simulink model "UNICO_simulink"  (R2023a)
settings: Solver=FixedStepAuto  StartTime=0.0  StopTime=750  RelTol=1e-3
undefined symbols (not defined in the file): Control, OutList, strmatch
libraries: cstblocks x3, simulink x2
settings Model: Creator=emanu  LastModifiedBy=utente
settings SolverCC: ZeroCrossAlgorithm=Adaptive
settings OptimizationCC: ReuseModelBlockBuffer=off
settings DebuggingCC: MaxConsecutiveZCsMsg=warning  IgnoredZcDiagnostic=none
settings ModelReferenceCC: EnableRefExpFcnMdlSchedulingChecks=on
settings RTWCC: Description=Create Visual C/C++ Solution File for Simulink Coder  SystemTargetFile=discon.tlc  TemplateMakefile=discon_vc.tmf
settings GRTTargetCC: UseToolchainInfoCompliant=off

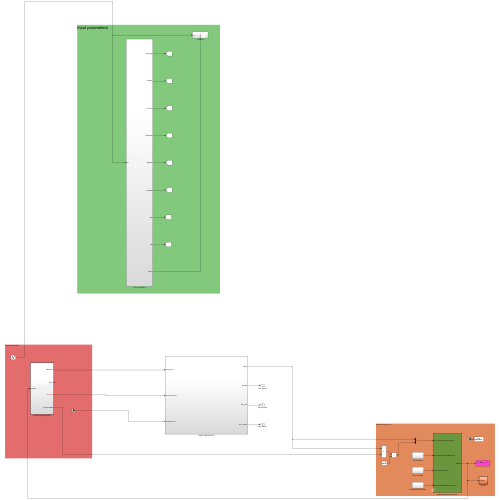
[thumbnail: Simulink's stored preview of the top-level diagram]
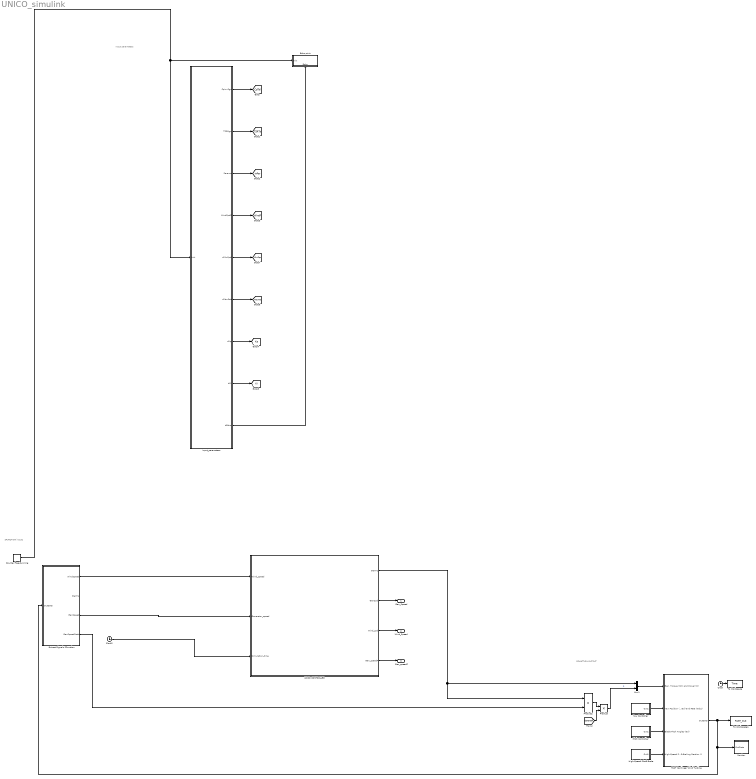
== system UNICO_simulink ==
  note: SFUNCTION inputs
  note: SFUNCTION OUTPUT
  note: Input parameters
  Clock : Clock
  Clock2 : Clock
  Counter Free-Running : simulink/Sources/Counter Free-Running  NumBits=64  tsamp=-1
  Echo print : Subsystem
      settings: PortSchema="{\"entries\":[{\"content\":{\"sides\":[{\"content\":{\"connectorIds\":[\"In1\"]},\"type\":\"ConnectorPlacement.EquallySpacedRectSide\",\"uuid\":\"a7404841-4279-4901-8e4b-4d9f651fd70d\"},{\"content\":{\"side\":\"RIGHT\"},\"type\":\"ConnectorPlacement.EquallySpacedRectSide\",\"uuid\":\"c083252d-994d-448b-85dd-b05fa098362a\"},{\"content\":{\"connectorIds\":[\"In2\"],\"side\":\"TOP\"},\"type\":\"ConnectorPlacement.EquallySpacedRectSide\",\"uuid\":\"2158789e-5709-45dd-87ec-c3c83921db3a\"}]},\"type\":\"ConnectorPlacement.EquallySpacedConnector\",\"uuid\":\"2f3f8f4d-3210-4d41-988d-02cc8661526f\"}],\"packageUris\":[\"http://schema.mathworks.com/mf0/Connector/R2020b\"],\"version\":\"1.0\"}"
  Extract Signals SFunction : Subsystem  TreatAsAtomicUnit=on
  FAST Nonlinear Wind Turbine : Subsystem  mask(FAST Nonlinear Wind Turbine){}
      mask help: This block contains the FAST S-Function.
      mask init:
      | clear FAST_SFunc
  High-Speed Shaft Brake : Subsystem
  Input_parameters : Subsystem
  Monitor : Subsystem  TreatAsAtomicUnit=on
  Mux1 : Mux  Inputs=2
  Pitch Controller : Subsystem
  Product : Product
  Product2 : Product
  To Workspace : ToWorkspace  VariableName=Time  SampleTime=-1
  To Workspace1 : ToWorkspace  VariableName=FAST_Out  SaveFormat=Timeseries  SampleTime=-1
  UNICO CONTROLLER : Subsystem
  Yaw Controller : Subsystem
  Gen_Speed : Outport
  Wind_Speed : Outport  Port=2
  Gen_speedF : Outport  Port=3
  tag scope: CpTbl=global, InPar=global, Ki=global, Kp=global, MaxRat=global, MinSpd=global, TSRTb=global, WindF=global
  wires:
  Pitch Controller/1(Out1) -> FAST Nonlinear Wind Turbine/3(Blade Pitch Angles (rad))
  High-Speed Shaft Brake/1(Out1) -> FAST Nonlinear Wind Turbine/4(High-Speed Shaft Braking Fraction (-))
  FAST Nonlinear Wind Turbine/1(OutData) -> Extract Signals SFunction/1(OutData), Monitor/1(OutData), To Workspace1/1
  Clock/1 -> To Workspace/1
  Yaw Controller/1(Out1) -> FAST Nonlinear Wind Turbine/2(Yaw Position (rad) and Rate (rad/s))
  Clock2/1 -> UNICO CONTROLLER/3(Simulation_time)
  Mux1/1 -> FAST Nonlinear Wind Turbine/1(Gen. Torque (Nm) and Power (W))
  Product2/1 -> Product/1
  Product/1 -> Mux1/2  "P"
  Input_parameters/9(dEcho) -> Echo print/2(Echo)
  Counter Free-Running/1 -> Echo print/1(Init), Input_parameters/1(Init)
  Input_parameters/2(TSRSgn) -> [TSRTb]
  Input_parameters/1(CpInvSgn) -> [CpTbl]
  Input_parameters/3(Params) -> [InPar]
  Input_parameters/4(WindSpdF) -> [WindF]
  Input_parameters/5(dMinSpd) -> [MinSpd]
  Input_parameters/6(dMaxRat) -> [MaxRat]
  Input_parameters/7(dKp) -> [Kp]
  Input_parameters/8(dKi) -> [Ki]
  [dGenEff] -> Product/2
  Extract Signals SFunction/1(WindSpeed) -> UNICO CONTROLLER/1(Wind_speed)
  Extract Signals SFunction/3(GenSpeed) -> UNICO CONTROLLER/2(Generator_speed)
  Extract Signals SFunction/4(GenSpeedRads) -> Product2/2
  UNICO CONTROLLER/1(GenTq) -> Mux1/1, Product2/1
  UNICO CONTROLLER/2(GenSpd) -> Gen_Speed/1
  UNICO CONTROLLER/3(Wind_spd) -> Wind_Speed/1
  UNICO CONTROLLER/4(Gen_speedF) -> Gen_speedF/1

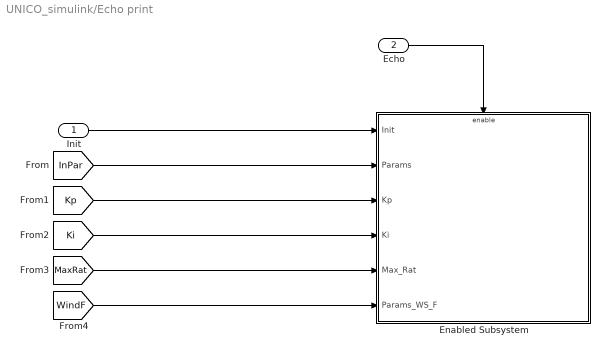
== system UNICO_simulink/Echo print ==
  Init : Inport
  Echo : Inport  Port=2
  Enabled Subsystem : Subsystem  TreatAsAtomicUnit=on
      settings: LibrarySourceBlock=|
      | hdlsllib/Ports &
      | Subsystems/Enabled
      | Subsystem
  wires:
  [InPar] -> Enabled Subsystem/2(Params)
  [Kp] -> Enabled Subsystem/3(Kp)
  [Ki] -> Enabled Subsystem/4(Ki)
  [MaxRat] -> Enabled Subsystem/5(Max_Rat)
  Init/1 -> Enabled Subsystem/1(Init)
  [WindF] -> Enabled Subsystem/6(Params_WS_F)
  Echo/1 -> Enabled Subsystem/Enable

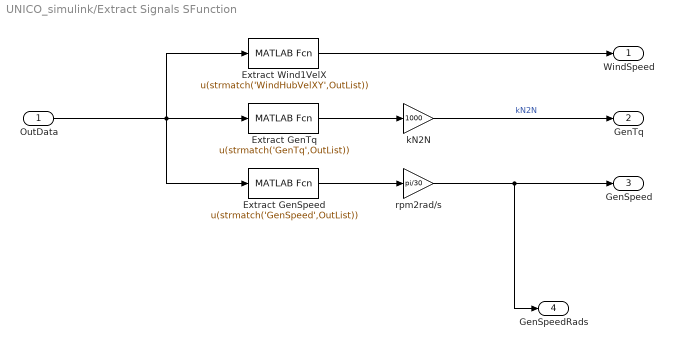
== system UNICO_simulink/Extract Signals SFunction ==
  OutData : Inport
  Extract GenSpeed : MATLABFcn  MATLABFcn=u(strmatch('GenSpeed',OutList))
  Extract GenTq : MATLABFcn  MATLABFcn=u(strmatch('GenTq',OutList))
  Extract Wind1VelX : MATLABFcn  MATLABFcn=u(strmatch('WindHubVelXY',OutList))
  kN2N : Gain  Gain=1000
  rpm2rad/s : Gain  Gain=pi/30
  WindSpeed : Outport  VectorParamsAs1DForOutWhenUnconnected=off
  GenTq : Outport  Port=2  VectorParamsAs1DForOutWhenUnconnected=off
  GenSpeed : Outport  Port=3  VectorParamsAs1DForOutWhenUnconnected=off
  GenSpeedRads : Outport  Port=4
  wires:
  Extract GenSpeed/1 -> rpm2rad/s/1
  OutData/1 -> Extract GenTq/1, Extract GenSpeed/1, Extract Wind1VelX/1
  kN2N/1 -> GenTq/1  "kN2N"
  Extract GenTq/1 -> kN2N/1
  rpm2rad/s/1 -> GenSpeedRads/1, GenSpeed/1
  Extract Wind1VelX/1 -> WindSpeed/1

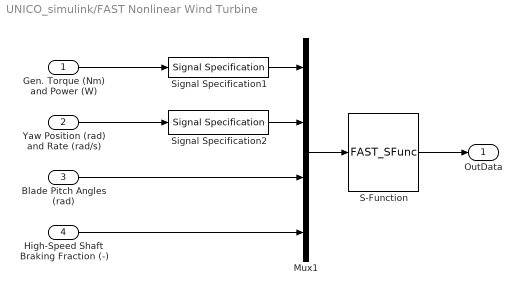
== system UNICO_simulink/FAST Nonlinear Wind Turbine ==
  Gen. Torque (Nm) and Power (W) : Inport
  Yaw Position (rad) and Rate (rad/s) : Inport  Port=2
  Blade Pitch Angles (rad) : Inport  Port=3
  High-Speed Shaft Braking Fraction (-) : Inport  Port=4
  Mux1 : Mux
  S-Function : S-Function  FunctionName=FAST_SFunc  Parameters=FAST_InputFileName, TMax, 0  SFunctionDeploymentMode=off  EnableBusSupport=off
  Signal Specification1 : SignalSpecification  OutDataTypeStr=double  Dimensions=2
  Signal Specification2 : SignalSpecification  OutDataTypeStr=double  Dimensions=2
  OutData : Outport
  wires:
  Gen. Torque (Nm) and Power (W)/1 -> Signal Specification1/1
  S-Function/1 -> OutData/1
  Mux1/1 -> S-Function/1
  Blade Pitch Angles (rad)/1 -> Mux1/3
  Yaw Position (rad) and Rate (rad/s)/1 -> Signal Specification2/1
  Signal Specification1/1 -> Mux1/1
  Signal Specification2/1 -> Mux1/2
  High-Speed Shaft Braking Fraction (-)/1 -> Mux1/4

== system UNICO_simulink/High-Speed Shaft Brake ==
  High-Speed Shaft Braking Fraction : Constant  Value=0
  Out1 : Outport
  wires:
  High-Speed Shaft Braking Fraction/1 -> Out1/1

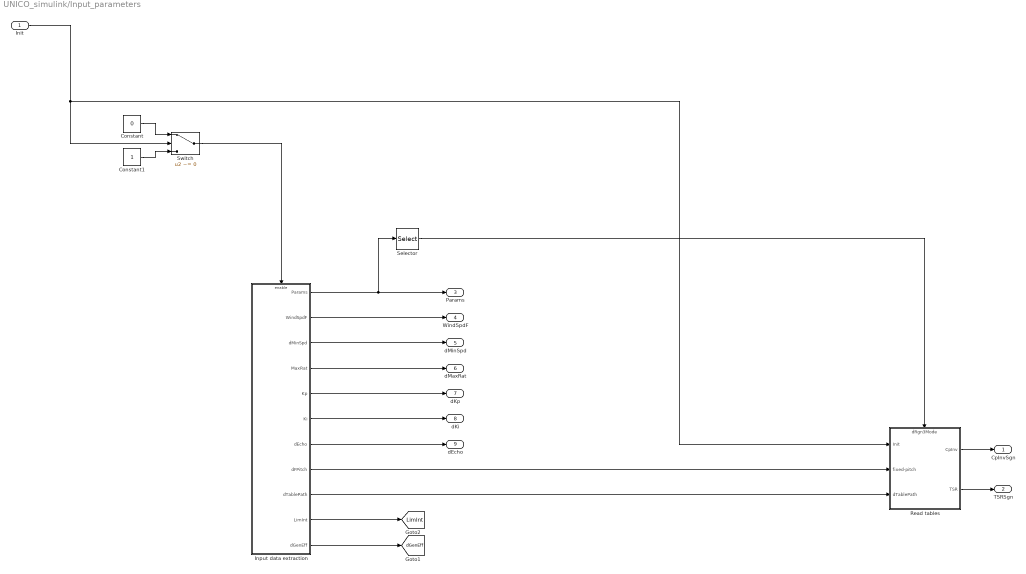
== system UNICO_simulink/Input_parameters ==
  Init : Inport
  Constant : Constant  Value=0
  Constant1 : Constant  SampleTime=-1
  Input data extraction : Subsystem  TreatAsAtomicUnit=on
      settings: LibrarySourceBlock=|
      | hdlsllib/Ports &
      | Subsystems/Enabled
      | Subsystem
  Read tables : Subsystem  TreatAsAtomicUnit=on
      settings: PortSchema="{\"entries\":[{\"content\":{\"sides\":[{\"content\":{\"connectorIds\":[\"In1\",\"In2\",\"In3\"]},\"type\":\"ConnectorPlacement.EquallySpacedRectSide\",\"uuid\":\"a7836439-e1fb-45be-ad70-3852da1eaa12\"},{\"content\":{\"connectorIds\":[\"Out1\",\"Out2\"],\"side\":\"RIGHT\"},\"type\":\"ConnectorPlacement.EquallySpacedRectSide\",\"uuid\":\"ffec095e-4721-408c-aa6b-05f74f8b0376\"},{\"content\":{\"connectorIds\":[\"In4\"],\"side\":\"TOP\"},\"type\":\"ConnectorPlacement.EquallySpacedRectSide\",\"uuid\":\"10a552ae-6062-490f-a1a4-19d2011a77e1\"}]},\"type\":\"ConnectorPlacement.EquallySpacedConnector\",\"uuid\":\"8ad70741-afb5-4f39-9da0-3165d0b94eda\"}],\"packageUris\":[\"http://schema.mathworks.com/mf0/Connector/R2020b\"],\"version\":\"1.0\"}"
      settings: LibrarySourceBlock=|
      | hdlsllib/Ports &
      | Subsystems/Enabled
      | Subsystem
  Selector : Selector  InputPortWidth=22  IndexOptions=Index vector (dialog)  Indices=[16]  OutputSizes=1
  Switch : Switch  Criteria=u2 ~= 0  SaturateOnIntegerOverflow=off  InputSameDT=off
  CpInvSgn : Outport
  TSRSgn : Outport  Port=2
  Params : Outport  Port=3
  WindSpdF : Outport  Port=4
  dMinSpd : Outport  Port=5
  dMaxRat : Outport  Port=6
  dKp : Outport  Port=7
  dKi : Outport  Port=8
  dEcho : Outport  Port=9
  tag scope: LimInt=global, dGenEff=global
  wires:
  Read tables/1(CpInv) -> CpInvSgn/1
  Read tables/2(TSR) -> TSRSgn/1
  Input data extraction/1(Params) -> Selector/1, Params/1
  Input data extraction/2(WindSpdF) -> WindSpdF/1
  Input data extraction/3(dMinSpd) -> dMinSpd/1
  Input data extraction/4(MaxRat) -> dMaxRat/1
  Input data extraction/5(Kp) -> dKp/1
  Input data extraction/6(Ki) -> dKi/1
  Input data extraction/7(dEcho) -> dEcho/1
  Input data extraction/8(dFPitch) -> Read tables/2(fixed-pitch)
  Input data extraction/9(dTablePath) -> Read tables/3(dTablePath)
  Constant1/1 -> Switch/3
  Constant/1 -> Switch/1
  Switch/1 -> Input data extraction/Enable
  Init/1 -> Switch/2, Read tables/1(Init)
  Input data extraction/10(LimInt) -> [LimInt]
  Input data extraction/11(dGenEff) -> [dGenEff]
  Selector/1 -> Read tables/4(dRgn3Mode)

== system UNICO_simulink/Monitor ==
  OutData : Inport
  Extract GenTq : MATLABFcn  MATLABFcn=u(strmatch('GenTq',OutList))
  Extract GenTq_1 : Fcn  Commented=on  Expr=u(strmatch('GenTq',OutList))
  Extract RotSpeed : MATLABFcn  MATLABFcn=u(strmatch('RotSpeed',OutList))
  Extract RotSpeed_1 : Fcn  Commented=on  Expr=u(strmatch('RotSpeed',OutList))
  Scope : Scope  NumInputPorts=2
  wires:
  OutData/1 -> Extract GenTq/1, Extract RotSpeed/1
  Extract RotSpeed/1 -> Scope/1
  Extract GenTq/1 -> Scope/2

== system UNICO_simulink/Pitch Controller ==
  Blade Pitch Angles : Constant  Value=zeros(1,3)'
  Out1 : Outport
  wires:
  Blade Pitch Angles/1 -> Out1/1

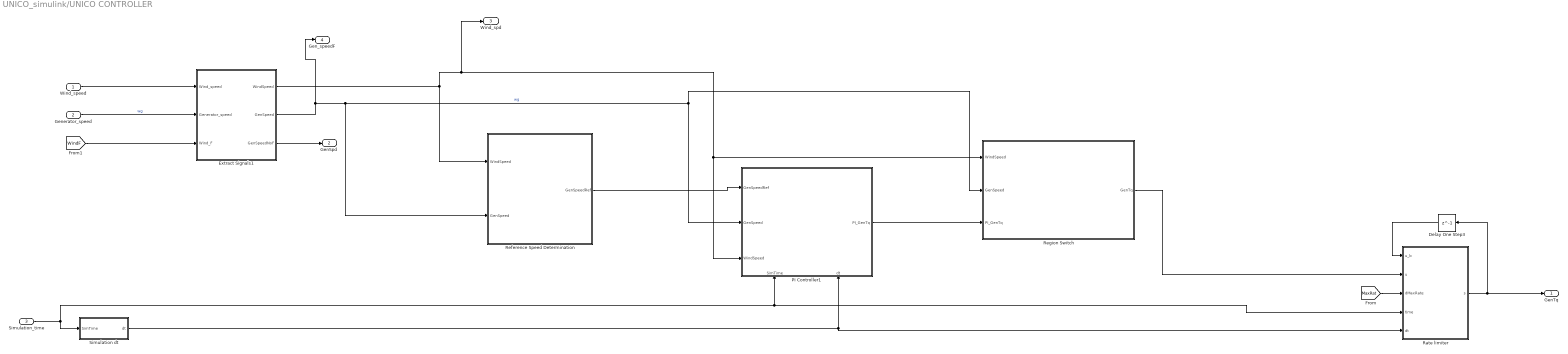
== system UNICO_simulink/UNICO CONTROLLER ==
  Wind_speed : Inport
  Generator_speed : Inport  Port=2
  Simulation_time : Inport  Port=3
  Delay One Step3 : Delay  DelayLength=1
  Extract Signals1 : Subsystem  TreatAsAtomicUnit=on
  PI Controller1 : Subsystem
      settings: PortSchema="{\"entries\":[{\"content\":{\"sides\":[{\"content\":{\"connectorIds\":[\"In1\",\"In2\",\"In3\"]},\"type\":\"ConnectorPlacement.EquallySpacedRectSide\",\"uuid\":\"bcfbec15-b5a6-4167-802a-412b097f843a\"},{\"content\":{\"connectorIds\":[\"Out1\"],\"side\":\"RIGHT\"},\"type\":\"ConnectorPlacement.EquallySpacedRectSide\",\"uuid\":\"a1a0e280-ec2e-4521-b7c2-616f76855769\"},{\"content\":{\"side\":\"TOP\"},\"type\":\"ConnectorPlacement.EquallySpacedRectSide\",\"uuid\":\"a387131f-be3d-4833-aaf7-26d744fefb98\"},{\"content\":{\"connectorIds\":[\"In4\",\"In5\"],\"side\":\"BOTTOM\"},\"type\":\"ConnectorPlacement.EquallySpacedRectSide\",\"uuid\":\"0ba6a37e-dab2-43ad-9644-c88e42fafd19\"}]},\"type\":\"ConnectorPlacement.EquallySpacedConnector\",\"uuid\":\"8b861741-8fda-4119-9715-572ab920b169\"}],\"packageUris\":[\"http://schema.mathworks.com/mf0/Connector/R2020b\"],\"version\":\"1.0\"}"
  Rate limiter : MATLAB Function  TreatAsAtomicUnit=on
  Reference Speed Determination : Subsystem
  "Region Switch " : Subsystem
  Simulation dt : Subsystem
  GenTq : Outport
  GenSpd : Outport  Port=2
  Wind_spd : Outport  Port=3
  Gen_speedF : Outport  Port=4
  wires:
  Extract Signals1/1(WindSpeed) -> Wind_spd/1, PI Controller1/3(WindSpeed), "Region Switch "/1(WindSpeed), Reference Speed Determination/1(WindSpeed)
  Simulation dt/1(dt) -> PI Controller1/5(dt), Rate limiter/5(dt)
  Extract Signals1/2(GenSpeed) -> Gen_speedF/1, Reference Speed Determination/2(GenSpeed), "Region Switch "/2(GenSpeed), PI Controller1/2(GenSpeed)  "wg"
  Generator_speed/1 -> Extract Signals1/2(Generator_speed)  "wg"
  Reference Speed Determination/1(GenSpeedRef) -> PI Controller1/1(GenSpeedRef)
  PI Controller1/1(PI_GenTq) -> "Region Switch "/3(PI_GenTq)
  Delay One Step3/1 -> Rate limiter/1(u_b)
  Simulation_time/1 -> Simulation dt/1(SimTime), Rate limiter/4(time), PI Controller1/4(SimTime)
  [MaxRat] -> Rate limiter/3(dMaxRate)
  Wind_speed/1 -> Extract Signals1/1(Wind_speed)
  Extract Signals1/3(GenSpeedNoF) -> GenSpd/1
  "Region Switch "/1(GenTq) -> Rate limiter/2(u)
  [WindF] -> Extract Signals1/3(Wind_F)
  Rate limiter/1(s) -> Delay One Step3/1, GenTq/1

== system UNICO_simulink/Yaw Controller ==
  Mux : Mux  Inputs=2
  Yaw Position : Constant  Value=0
  Yaw rate : Constant  Value=0
  Out1 : Outport
  wires:
  Mux/1 -> Out1/1
  Yaw Position/1 -> Mux/1
  Yaw rate/1 -> Mux/2

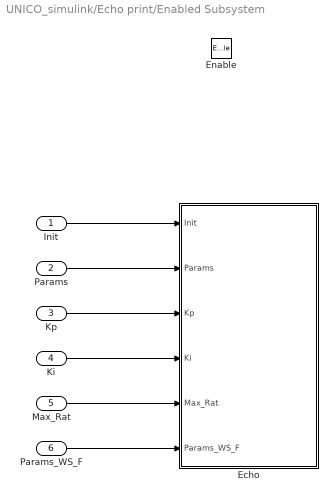
== system UNICO_simulink/Echo print/Enabled Subsystem ==
  Init : Inport
  Params : Inport  Port=2
  Kp : Inport  Port=3
  Ki : Inport  Port=4
  Max_Rat : Inport  Port=5
  Params_WS_F : Inport  Port=6
  Enable : EnablePort
  Echo : MATLAB Function  TreatAsAtomicUnit=on
  wires:
  Init/1 -> Echo/1(Init)
  Params_WS_F/1 -> Echo/6(Params_WS_F)
  Max_Rat/1 -> Echo/5(Max_Rat)
  Ki/1 -> Echo/4(Ki)
  Kp/1 -> Echo/3(Kp)
  Params/1 -> Echo/2(Params)

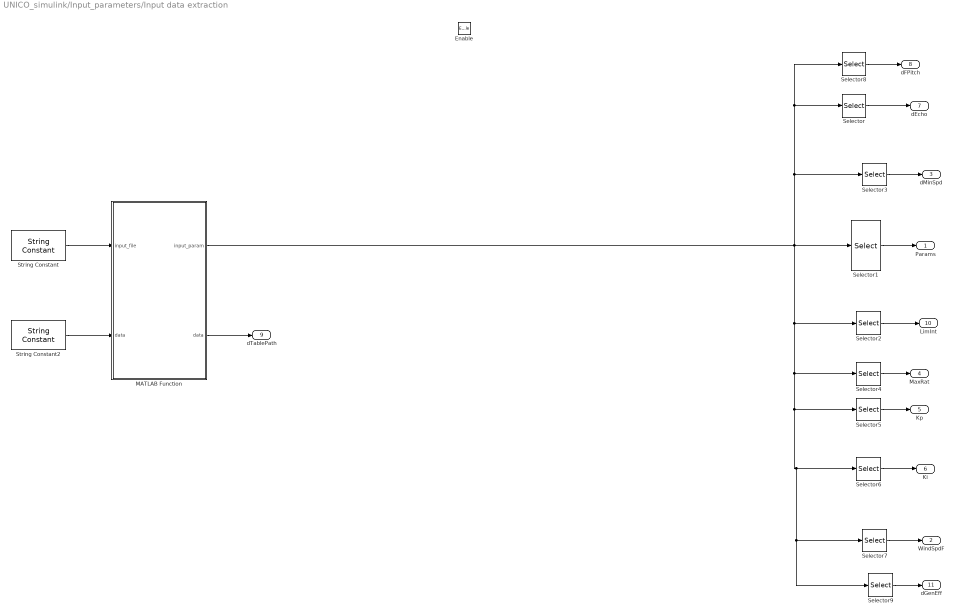
== system UNICO_simulink/Input_parameters/Input data extraction ==
  Enable : EnablePort
  MATLAB Function : MATLAB Function  TreatAsAtomicUnit=on
  Selector : Selector  InputPortWidth=31  IndexOptions=Index vector (dialog)  Indices=[1]  OutputSizes=1
  Selector1 : Selector  InputPortWidth=31  IndexOptions=Index vector (dialog)  Indices=[2 3 4 5 6 7 8 9 11 12 13 14 15 16 17 18 19 20 21 28 29 30]  OutputSizes=1
  Selector2 : Selector  InputPortWidth=31  IndexOptions=Index vector (dialog)  Indices=[4 8]  OutputSizes=1
  Selector3 : Selector  InputPortWidth=31  IndexOptions=Index vector (dialog)  Indices=[11]  OutputSizes=1
  Selector4 : Selector  InputPortWidth=31  IndexOptions=Index vector (dialog)  Indices=[10]  OutputSizes=1
  Selector5 : Selector  InputPortWidth=31  IndexOptions=Index vector (dialog)  Indices=[22]  OutputSizes=1
  Selector6 : Selector  InputPortWidth=31  IndexOptions=Index vector (dialog)  Indices=[23]  OutputSizes=1
  Selector7 : Selector  InputPortWidth=31  IndexOptions=Index vector (dialog)  Indices=[24 25 26 27]  OutputSizes=1
  Selector8 : Selector  InputPortWidth=31  IndexOptions=Index vector (dialog)  Indices=[31]  OutputSizes=1
  Selector9 : Selector  InputPortWidth=31  IndexOptions=Index vector (dialog)  Indices=[7]  OutputSizes=1
  String Constant : StringConstant  String=input_file
  String Constant2 : StringConstant  String="\"None\""
  Params : Outport
  WindSpdF : Outport  Port=2
  dMinSpd : Outport  Port=3
  MaxRat : Outport  Port=4
  Kp : Outport  Port=5
  Ki : Outport  Port=6
  dEcho : Outport  Port=7
  dFPitch : Outport  Port=8
  dTablePath : Outport  Port=9
  LimInt : Outport  Port=10
  dGenEff : Outport  Port=11
  wires:
  MATLAB Function/1(input_param) -> Selector9/1, Selector7/1, Selector6/1, Selector5/1, Selector4/1, Selector2/1, Selector8/1, Selector/1, Selector3/1, Selector1/1
  Selector1/1 -> Params/1
  Selector2/1 -> LimInt/1
  Selector3/1 -> dMinSpd/1
  String Constant/1 -> MATLAB Function/1(input_file)
  Selector9/1 -> dGenEff/1
  Selector8/1 -> dFPitch/1
  Selector5/1 -> Kp/1
  MATLAB Function/2(data) -> dTablePath/1
  Selector6/1 -> Ki/1
  Selector4/1 -> MaxRat/1
  Selector/1 -> dEcho/1
  Selector7/1 -> WindSpdF/1
  String Constant2/1 -> MATLAB Function/2("data ")

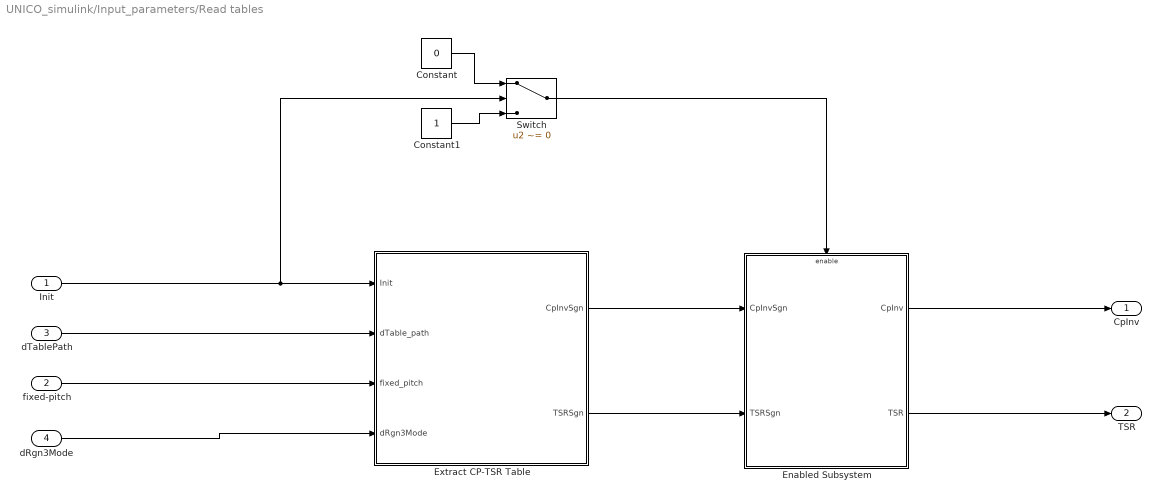
== system UNICO_simulink/Input_parameters/Read tables ==
  Init : Inport
  fixed-pitch : Inport  Port=2
  dTablePath : Inport  Port=3
  dRgn3Mode : Inport  Port=4
  Constant : Constant  Value=0
  Constant1 : Constant  SampleTime=-1
  Enabled Subsystem : Subsystem  TreatAsAtomicUnit=on
      settings: LibrarySourceBlock=|
      | hdlsllib/Ports &
      | Subsystems/Enabled
      | Subsystem
  Extract CP-TSR Table : MATLAB Function  TreatAsAtomicUnit=on
  Switch : Switch  Criteria=u2 ~= 0  Threshold=1  SaturateOnIntegerOverflow=off  InputSameDT=off
  CpInv : Outport
  TSR : Outport  Port=2
  wires:
  Constant1/1 -> Switch/3
  Enabled Subsystem/1(CpInv) -> CpInv/1
  Init/1 -> Switch/2, Extract CP-TSR Table/1(Init)
  Enabled Subsystem/2(TSR) -> TSR/1
  dTablePath/1 -> Extract CP-TSR Table/2(dTable_path)
  Switch/1 -> Enabled Subsystem/Enable
  Extract CP-TSR Table/2(TSRSgn) -> Enabled Subsystem/2(TSRSgn)
  Constant/1 -> Switch/1
  Extract CP-TSR Table/1(CpInvSgn) -> Enabled Subsystem/1(CpInvSgn)
  fixed-pitch/1 -> Extract CP-TSR Table/3(fixed_pitch)
  dRgn3Mode/1 -> Extract CP-TSR Table/4(dRgn3Mode)

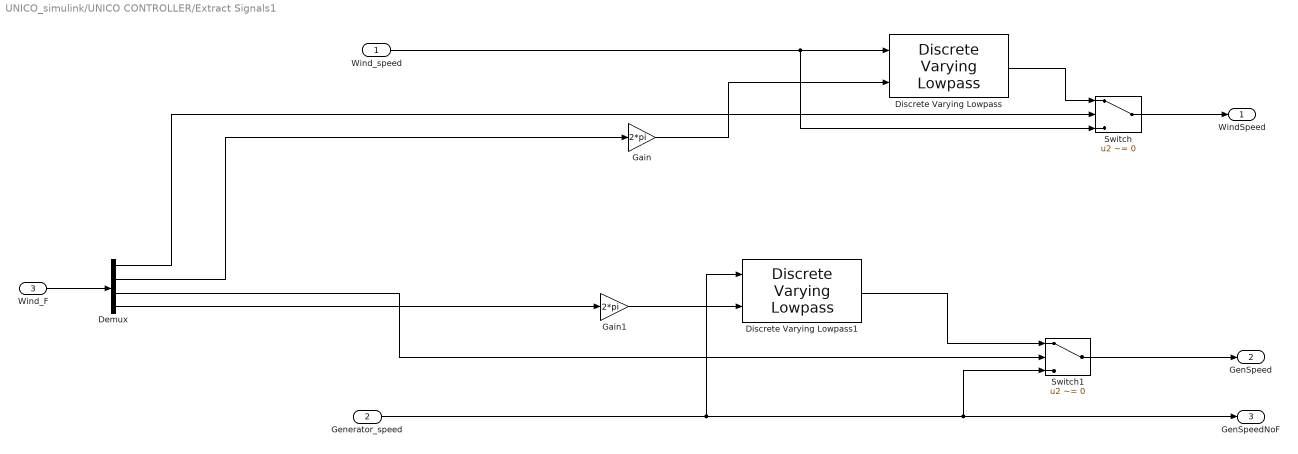
== system UNICO_simulink/UNICO CONTROLLER/Extract Signals1 ==
  Wind_speed : Inport
  Generator_speed : Inport  Port=2
  Wind_F : Inport  Port=3
  Demux : Demux
  Discrete Varying Lowpass : cstblocks/Linear Parameter Varying/Discrete Varying Lowpass  N=1  w0=0  Ts=Control.DT
  Discrete Varying Lowpass1 : cstblocks/Linear Parameter Varying/Discrete Varying Lowpass  N=1  w0=0  Ts=Control.DT
  Gain : Gain  Gain=2*pi
  Gain1 : Gain  Gain=2*pi
  Switch : Switch  Criteria=u2 ~= 0  SaturateOnIntegerOverflow=off  InputSameDT=off
  Switch1 : Switch  Criteria=u2 ~= 0  SaturateOnIntegerOverflow=off  InputSameDT=off
  WindSpeed : Outport  VectorParamsAs1DForOutWhenUnconnected=off
  GenSpeed : Outport  Port=2  VectorParamsAs1DForOutWhenUnconnected=off
  GenSpeedNoF : Outport  Port=3
  wires:
  Wind_speed/1 -> Switch/3, Discrete Varying Lowpass/1
  Generator_speed/1 -> Switch1/3, GenSpeedNoF/1, Discrete Varying Lowpass1/1
  Switch1/1 -> GenSpeed/1
  Discrete Varying Lowpass/1 -> Switch/1
  Demux/1 -> Switch/2
  Switch/1 -> WindSpeed/1
  Discrete Varying Lowpass1/1 -> Switch1/1
  Gain/1 -> Discrete Varying Lowpass/2
  Gain1/1 -> Discrete Varying Lowpass1/2
  Wind_F/1 -> Demux/1
  Demux/2 -> Gain/1
  Demux/3 -> Switch1/2
  Demux/4 -> Gain1/1

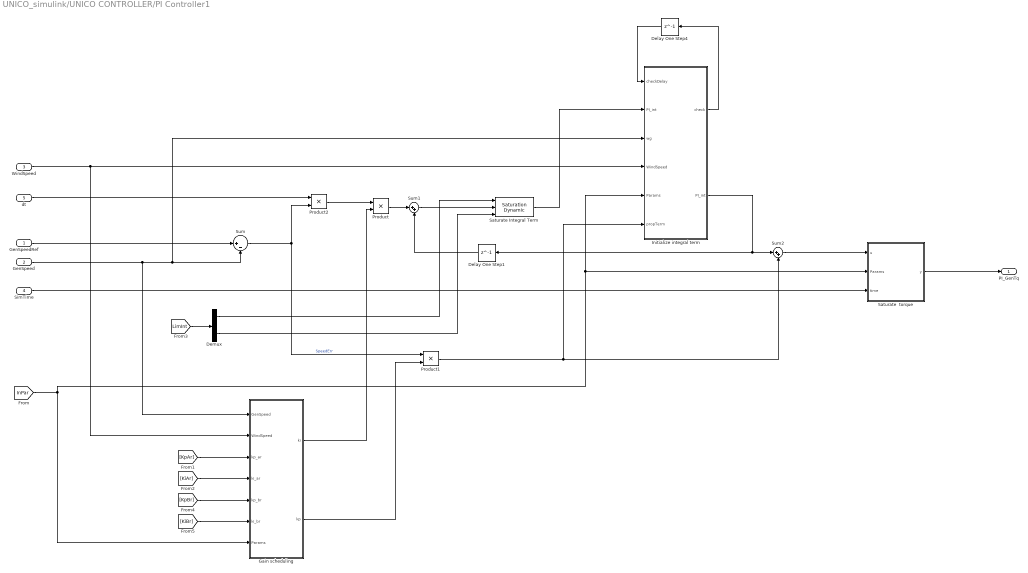
== system UNICO_simulink/UNICO CONTROLLER/PI Controller1 ==
  GenSpeedRef : Inport
  GenSpeed : Inport  Port=2
  WindSpeed : Inport  Port=3
  SimTime : Inport  Port=4
  dt : Inport  Port=5
  Delay One Step1 : Delay  DelayLength=1
  Delay One Step4 : Delay  DelayLength=1
  Demux : Demux  Outputs=2
  Gain scheduling : MATLAB Function  TreatAsAtomicUnit=on
  Initialize integral term : MATLAB Function  TreatAsAtomicUnit=on
  Product : Product
  Product1 : Product
  Product2 : Product
  Saturate  torque : MATLAB Function  TreatAsAtomicUnit=on
  Saturate Integral Term : simulink/Discontinuities/Saturation Dynamic  OutMin=[]  OutMax=[]  OutDataTypeStr=Inherit: Same as second input  OutDataType=fixdt(1, 16)  OutScaling=2^-10  RndMeth=Nearest  DoSatur=off
  Sum : Sum  Inputs=|+-
  Sum1 : Sum  Inputs=|++
  Sum2 : Sum  Inputs=|++
  PI_GenTq : Outport
  wires:
  GenSpeedRef/1 -> Sum/1
  GenSpeed/1 -> Gain scheduling/1(GenSpeed), Initialize integral term/3(wg), Sum/2
  Sum/1 -> Product2/2, Product1/1  "SpeedErr"
  Product/1 -> Sum1/1
  Product1/1 -> Sum2/2, Initialize integral term/6(propTerm)
  Sum1/1 -> Saturate Integral Term/2
  Saturate Integral Term/1 -> Initialize integral term/2("PI_int ")
  Product2/1 -> Product/1
  Delay One Step1/1 -> Sum1/2
  Demux/1 -> Saturate Integral Term/1
  Demux/2 -> Saturate Integral Term/3
  Sum2/1 -> Saturate  torque/1(u)
  Initialize integral term/1(check) -> Delay One Step4/1
  Delay One Step4/1 -> Initialize integral term/1(checkDelay)
  WindSpeed/1 -> Gain scheduling/2(WindSpeed), Initialize integral term/4(WindSpeed)
  Initialize integral term/2(PI_int) -> Delay One Step1/1, Sum2/1
  dt/1 -> Product2/1
  Saturate  torque/1(y) -> PI_GenTq/1
  [InPar] -> Initialize integral term/5(Params), Saturate  torque/2(Params), Gain scheduling/7(Params)
  Gain scheduling/2(kp) -> Product1/2
  Gain scheduling/1(ki) -> Product/2
  [LimInt] -> Demux/1
  SimTime/1 -> Saturate  torque/3(time)
  [KpAr] -> Gain scheduling/3(kp_ar)
  [KiAr] -> Gain scheduling/4(ki_ar)
  [KpBr] -> Gain scheduling/5(kp_br)
  [KiBr] -> Gain scheduling/6(ki_br)

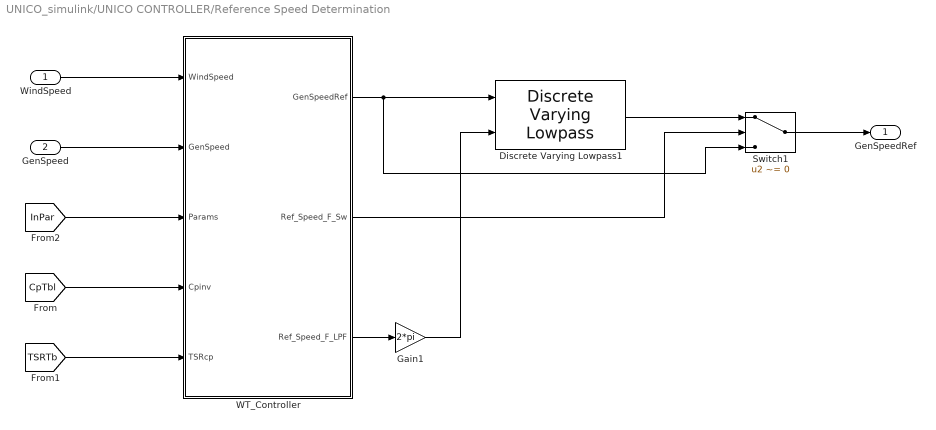
== system UNICO_simulink/UNICO CONTROLLER/Reference Speed Determination ==
  WindSpeed : Inport
  GenSpeed : Inport  Port=2
  Discrete Varying Lowpass1 : cstblocks/Linear Parameter Varying/Discrete Varying Lowpass  N=1  w0=0  Ts=Control.DT
  Gain1 : Gain  Gain=2*pi
  Switch1 : Switch  Criteria=u2 ~= 0  SaturateOnIntegerOverflow=off  InputSameDT=off
  WT_Controller : MATLAB Function  TreatAsAtomicUnit=on
  GenSpeedRef : Outport
  wires:
  WindSpeed/1 -> WT_Controller/1(WindSpeed)
  WT_Controller/1(GenSpeedRef) -> Switch1/3, Discrete Varying Lowpass1/1
  Gain1/1 -> Discrete Varying Lowpass1/2
  Switch1/1 -> GenSpeedRef/1
  Discrete Varying Lowpass1/1 -> Switch1/1
  WT_Controller/3(Ref_Speed_F_LPF) -> Gain1/1
  WT_Controller/2(Ref_Speed_F_Sw) -> Switch1/2
  [InPar] -> WT_Controller/3(Params)
  [CpTbl] -> WT_Controller/4(Cpinv)
  [TSRTb] -> WT_Controller/5(TSRcp)
  GenSpeed/1 -> WT_Controller/2(GenSpeed)

== system UNICO_simulink/UNICO CONTROLLER/Region Switch  ==
  WindSpeed : Inport
  GenSpeed : Inport  Port=2
  PI_GenTq : Inport  Port=3
  Region 2 Switch Mode : MATLAB Function  TreatAsAtomicUnit=on
  GenTq : Outport
  wires:
  WindSpeed/1 -> Region 2 Switch Mode/1(WindSpeed)
  GenSpeed/1 -> Region 2 Switch Mode/2(GenSpeed)
  PI_GenTq/1 -> Region 2 Switch Mode/3(PI_GenTq)
  Region 2 Switch Mode/1(GenTq) -> GenTq/1
  [InPar] -> Region 2 Switch Mode/4(Params)

== system UNICO_simulink/UNICO CONTROLLER/Simulation dt ==
  SimTime : Inport
  Delay One Step2 : Delay  DelayLength=1
  Sum3 : Sum  Inputs=|+-
  dt : Outport
  wires:
  Delay One Step2/1 -> Sum3/2
  SimTime/1 -> Delay One Step2/1, Sum3/1
  Sum3/1 -> dt/1

== system UNICO_simulink/Input_parameters/Read tables/Enabled Subsystem ==
  CpInvSgn : Inport
  TSRSgn : Inport  Port=2
  Enable : EnablePort
  CpInv : Outport
  TSR : Outport  Port=2
  wires:
  CpInvSgn/1 -> CpInv/1
  TSRSgn/1 -> TSR/1

== matlab function UNICO_simulink/Echo print/Enabled Subsystem/Echo ==
  data: Init input; Params input; Kp input; Ki input; Max_Rat input; Params_WS_F input
function fcn(Init, Params, Kp, Ki, Max_Rat, Params_WS_F)

R               = Params(1);  % Rotor radius [m]
v_rt            = Params(2);  % Rated wind speed  [m/s]
Rt_Tq           = Params(3);  % Rated torque  [Nm]
Pt              = Params(4);  % Rated Power [-]
w_rt            = Params(5);  % Rated Geerator Speed  [W]
eta             = Params(6);  % Generator Efficiency [-]
Min_Tq          = Params(7); % Minimum Torque [Nm]
Max_Tq          = Params(8);  % Maximum torque  [Nm]
w_min           = Params(9);  % Minimum generator speed  [rad/s]
r2              = Params(10);    % Region 2 control mode [-]
KSwitch         = Params(11);  % Switch for user defined k [-] 
Rgn2K           = Params(12);    %user defined K value [Nms^2/rad^2] 
SpdSwitch       = Params(13);  % velocity switch between Rgn 2 and 2 1/2 [rad/s]
TSR_opt         = Params(14);   %optimal TSR [-]
w_minSwitch     = Params(15); % Velocity switch between Rgn 1.5 and 2 [rad/s]
Cpmax           = Params(16);     % Optimal Cp [-]
r3              = Params(17);  % Region 3 control mode [-]
m               = Params(18);  % Angular coefficient Region 3 linear method
V_lin           = Params(19);  % Wind speed to start linear reduction [m/s]
Ref_Speed_F_Sw  = Params(20); % Reference speed filter switch [-]
Ref_Speed_F_LPF = Params(21); % Reference speed cut-off frequency [Hz]
rho             = Params(22);  % Air density             [kg/m^3]
Wind_Speed_F_Sw = Params_WS_F(1); % switch for wind speed Low-pass filter [-]
Wind_Speed_F_LPF= Params_WS_F(2); % wind speed low pass filter frequency [Hz]
Gen_Speed_F_Sw  = Params_WS_F(3); % Switch for generator speed low-pass filter [-]
Gen_Speed_F_LPF = Params_WS_F(4); % Generator speed low pass frequeny [Hz]




if Init == 0
    
f_echo = fopen('UNICO_echo.txt','w');
fprintf(f_echo,'UNICO CONTROLLER SIMULATION INPUT \n');
fprintf(f_echo,'Rotor radius [m]:                           %f \n',R);
fprintf(f_echo,'Rated wind speed [m/s]:                     %f \n',v_rt);
fprintf(f_echo,'Rated Torque [Nm]:                          %f \n',Rt_Tq);
fprintf(f_echo,'Rated power [W]:                            %f \n',Pt);
fprintf(f_echo,'Rated generator speed [rad/s]:              %f \n',w_rt);
fprintf(f_echo,'Generator efficiency [-]:                   %f \n',eta);
fprintf(f_echo,'Minimum Torque [Nm]:                        %f \n',Min_Tq);
fprintf(f_echo,'Maximum generator torque [Nm]:              %f \n',Max_Tq);
fprintf(f_echo,'Maximum generator torque rate [Nm/s]:       %f \n',Max_Rat);
fprintf(f_echo,'Minumum generator speed [rad/s]:            %f \n',w_min);
fprintf(f_echo,'Switch between Rgn1.5 and 2 [rad/s]:        %f \n',w_minSwitch);
fprintf(f_echo, 'Region 2 control [-]:                      %f \n', r2);
fprintf(f_echo,'Switch for user defined K [-]:              %f \n',KSwitch);
fprintf(f_echo,'User defined K value [Nms^2/rad^2]:         %f \n',Rgn2K);
fprintf(f_echo,'Switch between Rgn2 and 2.5 [rad/s]:        %f \n',SpdSwitch);
fprintf(f_echo,'Optimum TSR [-]:                            %f \n',TSR_opt);
fprintf(f_echo,'Maximum Cp value [-]:                       %f \n', Cpmax);
fprintf(f_echo,'Region 3 control [-]:                       %f \n',r3);
fprintf(f_echo,'Angular coefficient linear method []:       %f \n',m);
fprintf(f_echo,'Start reduction of ref velocity [m/s]:      %f \n', V_lin);
fprintf(f_echo,'PI Controller Kp [Nms/rad]:                 %f \n',Kp);
fprintf(f_echo,'PI Controller Ki [Nm/rad]:                  %f \n',Ki);
fprintf(f_echo,'Switch Wind speed filter [-]:               %f \n',Wind_Speed_F_Sw);
fprintf(f_echo,'Wind speed lowpass frequency[Hz]:           %f \n',Wind_Speed_F_LPF);
fprintf(f_echo,'Switch Generator speed filter [-]:          %f \n',Gen_Speed_F_Sw);
fprintf(f_echo,'Generator speed lowpass frequency [Hz]:     %f \n',Gen_Speed_F_LPF);
fprintf(f_echo,'Switch reference speed filter [-]:          %f \n',Ref_Speed_F_Sw);
fprintf(f_echo,'Reference speed lowpass frequency [Hz]:     %f \n',Ref_Speed_F_LPF);
fprintf(f_echo,'Air density [kg/m^3]:                       %f \n',rho);
fclose(f_echo);

end

== matlab function UNICO_simulink/Input_parameters/Read tables/Extract CP-TSR Table ==
  settings: updateMethod=DISCRETE
  data: Init input; dTable_path input; CpInvSgn output size=[513 1]; TSRSgn output size=[513 1]; fixed_pitch input; dRgn3Mode input
function [ CpInvSgn, TSRSgn] = fcn(Init, dTable_path, fixed_pitch, dRgn3Mode)

if Init == 0 && dRgn3Mode == 0  % if it is the first time we run the simulation and we need to extract the data (Optimum TSR tracking in Region 3)
    % extract the path from the input file
    aux = extractBefore(dTable_path,'!');
    RotPerfFile = strtrim(aux); % remove additional spaces at the end of the string

    fid = fopen(RotPerfFile, 'r');  % open table file
    if fid == -1

        error('Error loading file')
    end

    % Read first line to start tline
    tline = fgetl(fid);
    %initialize counters and variables. maximum allowed table size is
    %100x100
    % maximum number of pitch angles is 100
    count = 0;
    count_line = 1;
    TSR = zeros(1,100);
    Cp = zeros(100,100);
    pitch = zeros(1,100);
    % read through the file
    while ~feof(fid)

        tline = fgetl(fid);
       
        if isempty(tline) % skip empty lines
            count = count + 1;
            count_line = 1;

        elseif strcmp(tline(1),'#') % skip lines starting with #


            count = count + 1;
            count_line = 1;

        else  

            if count == 3 % the third part of the input file contains the pitch angles for the TSR-CP data
                idxs = isspace(tline);
                count_val = 1;
                count_in = 1;
                for i = 1:length(tline)
                    if idxs(i)==1
                        if idxs(i-1)==0


                            val = tline(count_in:i-1);
                            pitch(count_val) = real(str2double(val)); % extract the pitch data
                            count_val = count_val +1;
                        else
                            count_in = i;
                        end

                    end

                end



            elseif count == 4  % the fourth part of the file contains the TSR values
                % TSR Array
                idxs = isspace(tline);
                count_val = 1;
                count_in = 1;
                for i = 1:length(tline)
                    if idxs(i)==1
                        if idxs(i-1)==0


                            val = tline(count_in:i-1);
                            TSR(count_val) = real(str2double(val)); % store TSR values
                            count_val = count_val +1;
                        else
                            count_in = i;
                        end

                    end

                end


            elseif count == 8  % the fifth part of the file contains the CP values

                % Cp matrix
                idxCp = isspace(tline);
                count_val = 1;
                count_in = 1;
                for i = 1:length(tline)
                    if idxCp(i)==1
                        if idxCp(i-1)==0


                            val = tline(count_in:i-1);
                            Cp(count_line,count_val) = real(str2double(val)); % store cp values
                            count_val = count_val +1;
                        else
                            count_in = i;
                        end

                    end

                end
                count_line = count_line+1;
            end


        end

    end
    
    % locate the wanted pitch values
    AngleInd = find(pitch==fixed_pitch);
    CpInv1 = Cp(:,AngleInd(1));  % extract the data at the wanted pitch angle

    % initialize variables
    Cpmax = 0;
    maxind = 0;
    [Cpmax,maxind] = max(CpInv1);   % Extract maximum power coefficient value and its array index
  
   
    CpInv = zeros(maxind,1);
    CpInv(1:maxind,:) = CpInv1(1:maxind,:); % store the part of the CP curve that can be inverted for the TSR tracking strategy in region 3
    
    TSRcp = zeros(1,maxind);

    TSRcp(1,1:maxind) = TSR(1,1:maxind); % store corresponding TSR values

    % flip the arrays
    TSRSgn = TSRcp';  
    CpInvSgn = CpInv;  

else
  % if we have already read the table or we do need it
    TSRSgn = 0;  

    CpInvSgn= 0;
    
end

== matlab function UNICO_simulink/UNICO CONTROLLER/Region Switch /Region 2 Switch Mode ==
  data: WindSpeed input; GenSpeed input; PI_GenTq input; GenTq output; Params input
function GenTq = Rgn2_Fcn(WindSpeed, GenSpeed, PI_GenTq, Params)

% Load R struct variables
R       = Params(1);  % Rotor radius           [m]
v_rt    = Params(2);  % Rated power wind speed [m/s]
w_rt    = Params(5);  % Rated generator speed  [rad/s]
w_min   = Params(9);  % Minimum generator speed            [rad/s]
r2      = Params(10);  % Region 2 control mode  {0: optimum tsr tracking; 1: kw^2 torque law}
KSwitch = Params(11); % switch for user defined k
Rgn2K = Params(12); % user defined k {used only if KSwitch = 1}
SpdSwitch = Params(13); % speed switch from region 2 to 2 2 1/2
w_minSwitch = Params(14); % Switch between region 1.5 and 2 [rad/s]
TSR_opt = Params(15);  % Optimum TSR            [-]
Cpmax = Params(16);   % max cp value [-]
rho     = Params(22);  % Air density            [kg/m^3]



% Define parameters
wg  = GenSpeed;
v   = WindSpeed;
if KSwitch == 1
    K = Rgn2K;
else
    K   = 0.5*rho*pi*R^5*Cpmax/TSR_opt^3;  % K coefficient
end
w1  = SpdSwitch; % switching rotational speed for region 2.5 to 3
Tg1 = K*w1^2;   % torque value at the switching rotational speed
w2 = w_minSwitch;  % switching rotational speed for region 1.5 to 2
Tg2 = K*(w2)^2; % generator torque at the switching rotational speed from k-w^2 law
Tgmin = K*w_min^2; % generator torque at minimum rotational speed from k-w^2 law

% kw^2 control mode
if r2 == 1

    % if we are in region 1.5 or 2
    if (wg < w1) && (v <= v_rt)
        % use k-w^2 law
        GenTq =  K*wg^2;
        if wg < w2 % if the generator speed is smaller than the 1.5 switching value
            if PI_GenTq < Tg2 && PI_GenTq > Tgmin

                % use linear interpolation to smooth the switch between the two
                % regions
                GenTq = Tg2+(PI_GenTq-Tg2)/(w_min-w2)*(wg-w2);
               
            elseif PI_GenTq < Tgmin

                % in region 1.5 use TSR tracking to track the minimum speed
                % defined by the user
                GenTq = PI_GenTq;
                
            end
        end

    elseif (wg < w_rt) && (v <= v_rt)
        % region 2.5, smoothing of switch between region 2 and 3
        GenTq = Tg1+(PI_GenTq-Tg1)/(w_rt-w1)*(wg-w1);
    else
        % region 3
        GenTq = PI_GenTq;
    end
    % tsr tracking control mode
else
    GenTq = PI_GenTq;
end

== matlab function UNICO_simulink/UNICO CONTROLLER/PI Controller1/Gain scheduling ==
  data: GenSpeed input; WindSpeed input; kp_ar input; ki output; ki_ar input; kp_br input; ki_br input; kp output; Params input
function [ki,kp] = fcn(GenSpeed, WindSpeed, kp_ar, ki_ar,kp_br, ki_br, Params)

R       = Params(1);  % Rotor radius           [m]
v_rt    = Params(2);  % Rated power wind speed [m/s]
w_rt    = Params(5);  % Rated generator speed  [rad/s]
r2      = Params(10);  % Region 2 control mode  {0: optimum tsr tracking; 1: kw^2 torque law}
SpdSwitch = Params(13); %generator speed for switch between region 2 and 2 1/2

% if we use TSR tracking in below rated conditions, schedule the PI
% coefficients
if r2 == 0

    if WindSpeed < v_rt && GenSpeed < w_rt

        % if GenSpeed <=SpdSwitch
        if GenSpeed <= SpdSwitch
            kp = kp_br;
            ki = ki_br;

        elseif GenSpeed > SpdSwitch && GenSpeed <w_rt
            % else

            kp = kp_br+(kp_ar-kp_br)/(w_rt-SpdSwitch)*(GenSpeed-SpdSwitch);
            ki = ki_br+(ki_ar-ki_br)/(w_rt-SpdSwitch)*(GenSpeed-SpdSwitch);

        else

            kp = kp_ar;
            ki = ki_ar;
            % end
        end


    else

        kp = kp_ar;
        ki = ki_ar;
    end

else
    % if k-w is used only a set of kp and ki is used
    kp = kp_ar;
    ki = ki_ar;

end

== matlab function UNICO_simulink/Input_parameters/Input data extraction/MATLAB Function ==
  data: input_file input; input_param output; data input; data output
function [input_param,data]    = fcn(input_file, data)
%#read input data - this function is different when simulink or dll are
%used
%% read input data


% initialize input_param array
input_param = zeros(31,1);
% initialize table path
dTablePath = '';
% open input file
f_in = fopen(input_file);
count_p = 1;

while ~feof(f_in)


    tline = fgetl(f_in);

    if isempty(tline) % skip empty lines


    elseif strcmp(tline(1),'#') % skip lines starting with #

    

    else

        aux = extractBefore(tline,'!'); % extract data befor ! character
        str = strtrim(aux);    % trim unwanted spaces in the txt file

        num = real(str2double(str));  % convert string to double
        if isnan(num)  % if the output is nan, the value is not a number but we have reached the path to the TSR-CP table
            if input_param(19) == 0   % if we do  need the TSR-CP talbe
                str = tline; % extract the table path
                dTablePath = str;

            else  % if we do not need the path store none in the variable
                dTablePath = 'None';

            end

        else % if parameter is a number
            
            input_param(count_p) = num;  % store parameter in the variable and count 
            count_p = count_p +1;

        end
       
        
    end


end

fclose(f_in); % close input_data file
data = convertCharsToStrings(dTablePath); % convert the path to string for data transfer to other blocks

== matlab function UNICO_simulink/UNICO CONTROLLER/PI Controller1/Initialize integral term ==
  data: checkDelay input; check output; PI_int input; PI_int output; wg input; WindSpeed input; Params input; propTerm input
function [check,PI_int] = fcn(checkDelay, PI_int, wg,WindSpeed,Params, propTerm)

% Load R struct variables

R       = Params(1);  % Rotor radius           [m]
v_rt    = Params(2);  % Rated power wind speed [m/s]
w_rt    = Params(5);  % Rated generator speed  [rad/s]
w_min   = Params(9);  % Minimum generator speed            [rad/s]
r2      = Params(10);  % Region 2 control mode  {0: optimum tsr tracking; 1: kw^2 torque law}
KSwitch = Params(11); % Region 2 K- switch
Rgn2K = Params(12);   % user defined K value
SpdSwitch = Params(13); %generator speed for switch between region 2 and 2 1/2
w_minSwitch = Params(14); % Switch between region 1.5 and 2 [rad/s]
TSR_opt = Params(15);  % Optimum TSR            [-]
Cpmax   = Params(16); % max cp value [-]

rho     = Params(22);  % Air density            [kg/m^3]


if r2 == 1
    w1  = SpdSwitch;
    if KSwitch == 1
        K = Rgn2K;
    else
        K   = 0.5*rho*pi*R^5*Cpmax/TSR_opt^3;  % K coefficient
    end
    if (wg < w1) && (WindSpeed <= v_rt)
        % region 2. Store idx to check at following time step
        if wg< w_minSwitch
            % Region 1.5 We have to evaluate if we need to initialize the
            % integral term
            check = 0;
            if checkDelay == 2 % we are coming from region 2, initialize to the k-w^2 value at wg = w1
                
                Tg1 = K*wg^2; % torque value from k-w^2 law
                PI_int = (Tg1)-propTerm;  %initialize integral term
            elseif checkDelay == 0
                % we were already in Region 1.5
                % do not initialize Integral term

            end

        else
            % we are in region 2
            check = 2; 

        end

    elseif (wg < w_rt) && (WindSpeed<=v_rt) % we are in 2 1/2
        %region 2 1/2. We have to evaluate if we we need to initialize the
        %integral term
        check = 1;

        if checkDelay == 2 % we are coming from region 2, initialize to the k-w^2 value at wg = w1

            Tg1 = K*wg^2; % torque value from k-w^2 law
            PI_int = (Tg1)-propTerm;  %initialize integral term


        elseif checkDelay == 3

            %when coming from region 3 do not modify integral term, we are
            %already using PI controller
            
        else


            % do not modify integral term, checkDelay = 1 -> PI controller
            % already running. 
        end


    else
        % if we are in region 3  Store variable check to identify when we go back to region 2 1/2.
        check = 3;


    end

else
    % do not do anything, region 2 uses a PI controller.
    check = 0;

end

== matlab function UNICO_simulink/UNICO CONTROLLER/PI Controller1/Saturate  torque ==
  data: u input; y output; Params input; time input
function y = fcn(u,Params, time)


Min_Tq = Params(7);  %minimum torque value  [Nm]
Max_Tq = Params(8);  % maximum torque value  [Nm]

if time < 20   % at the beginning of the simulation do not apply torque saturation to avoid divergence
    y = u;
else

    if u > Max_Tq  % if torque from controller is larger than maximum saturation value
        

        y = Max_Tq;  % set the torque value to the MaxTq

    elseif u < Min_Tq  % if torque from controller is smaller than minimum saturation value

        y = Min_Tq;  % set torque value to MinTq

    else   % if torque from controller is within the max and min values, do not modify the output torque value

        y = u;


    end
end

== matlab function UNICO_simulink/UNICO CONTROLLER/Rate limiter ==
  data: u_b input; u input; s output; dMaxRate input; time input; dt input
function s = fcn(u_b,u,dMaxRate, time, dt)
% rate limiter applied only after 20 seconds to allow for controller
% initialization
if time>20
    rate_lim_pos = dMaxRate; % rate limit for torque is simmetric
    rate_lim_neg = -dMaxRate;
    % calculate torque rate
    rate = (u-u_b)/dt;

    if rate > rate_lim_pos % if the torque rate is larger than the maximum allowed, set the torque using the maximum rate

        u = u_b+rate_lim_pos*dt;

    elseif rate < rate_lim_neg % if the torque rate is smaller than the minimum allowed, set the torque using the minimum rate

        u = u_b+rate_lim_neg*dt;

    end

else

end
% if the maximum torque rate is not violated
s = u;

== matlab function UNICO_simulink/UNICO CONTROLLER/Reference Speed Determination/WT_Controller ==
  data: WindSpeed input; GenSpeed input; GenSpeedRef output; Params input; Cpinv input; TSRcp input; Ref_Speed_F_Sw output; Ref_Speed_F_LPF output
function [GenSpeedRef, Ref_Speed_F_Sw,Ref_Speed_F_LPF]  = WT_Controller(WindSpeed, GenSpeed, Params, Cpinv, TSRcp)

% Load struct variables
R       = Params(1);  % Rotor radius            [m]
v_rt    = Params(2);  % Rated wind speed   [m/s]
Pt      = Params(4);  % RatedPwr             [W]
w_rt    = Params(5);  % RatedGenSpeed             [rad/s]
eta     = Params(6);  % Generator Efficiency [-]
w_min   = Params(9);  % Minimum generator speed            [rad/s]
r2      = Params(10);    % Region 2 control mode [-]
TSR_opt = Params(15);   %optimal TSR [-]
Cpmaxval= Params(16); % max CP value [-]
r3      = Params(17);  % Region 3 control mode [-]
m       = Params(18);  % Angular coefficient Region 3 linear method []
V_lin   = Params(19);  % Wind speed to start linear reduction [m/s]
Ref_Speed_F_Sw = Params(20); % Reference speed filter switch [-]
Ref_Speed_F_LPF = Params(21); % Reference speed cut-off frequency [Hz]
rho     = Params(22);  % Air density             [kg/m^3]


% Define parameters
v       = WindSpeed;   % Reassign parameter
w_opt   = v*TSR_opt/R; % Optimum generator speed (corresponding to optimum TSR)

% Region 1/Region 2 /Region 2 1/2
if v <= v_rt
    if r2 == 0
        w_ref = min(max(w_min,w_opt),w_rt);  
    else
        % for switching region
        if abs(w_rt-GenSpeed)<abs(w_min-GenSpeed)
            %region 2.5
            w_ref = w_rt;
        else
            % region 1.5
            w_ref = w_min;

        end

    end
       
% Region 3
else
    % Rated power tracking
    if r3 == 0
     
        Cp    = Pt*eta/(0.5*rho*pi*R^2*v^3);
        Cp    = min(max(0,Cp),Cpmaxval);
        TSR   = interp1(Cpinv,TSRcp,Cp);
        w_ref = TSR*v/R;

    else %linear reduction 
        
        if v< V_lin
            w_ref = w_rt;
        else
            w_ref = w_rt+m*(v-V_lin);
            w_ref = max(w_ref,w_min);

        end
    end
end

GenSpeedRef = w_ref;  % PI controller reference rotational speed
